simulink model "Perfect_Lineaer"  (R2017a)
settings: Solver=VariableStepAuto  StartTime=0.0  StopTime=17  FixedStep=0.01  RelTol=1e-3
values from neighbouring files (symbols this model uses):
  A = [-4.65E-06	0.0001701	-0.0002836	0	0	0	-2.56E-06	-7.97E-06	3.61E-06 ... (first row only)    [surfaces_setup_test.m]
  A0 = [-4.65E-06	0.0001701	-0.0002836	0	0	0	0	-1.43	0 ... (first row only)    [surfaces_setup_test.m]
  a0_s2345 = [0;0;0.05;0.05]    [HW5_4_surfaces.m]    (also in TEST_aerosetup.m; surfaces_setup_test.m)
  A_2345 = c_2345.*b_2345    [HW5_4_surfaces.m]    (also in TEST_aerosetup.m; surfaces_setup_test.m)
  Aileron_left = 0    [HW5_4_surfaces.m]    (also in TEST_aerosetup.m; surfaces_setup_test.m)
  Aileron_right = 0    [HW5_4_surfaces.m]    (also in TEST_aerosetup.m; surfaces_setup_test.m)
  B = [-7.98E-09	7.83E-09	1.68E-09	2.75E-10 ... (first row only)    [surfaces_setup_test.m]
  B0 = [-6.2	6.2	0	0.45 ... (first row only)    [surfaces_setup_test.m]
  c_2345 = [0.075;0.08;0.1;0.1]    [HW5_4_surfaces.m]    (also in TEST_aerosetup.m; surfaces_setup_test.m)
  CD0_s2345 = [0.01;0.01;0.01;0.01]    [HW5_4_surfaces.m]    (also in TEST_aerosetup.m; surfaces_setup_test.m)
  CDa_s2345 = [1;1;1;1]    [HW5_4_surfaces.m]    (also in TEST_aerosetup.m; surfaces_setup_test.m)
  CL0_2345 = [0;0; 0.05; 0.05]    [HW5_4_surfaces.m]    (also in TEST_aerosetup.m; surfaces_setup_test.m)
  CLa = 2*pi*(r./(2+r))    [HW5_4_surfaces.m]    (also in TEST_aerosetup.m; surfaces_setup_test.m)
  CM0_s2345 = [0;0;-0.05;-0.05]    [HW5_4_surfaces.m]    (also in TEST_aerosetup.m; surfaces_setup_test.m)
  CMa_s2345 = [0; 0; 0; 0]    [HW5_4_surfaces.m]    (also in TEST_aerosetup.m; surfaces_setup_test.m)
  e_s2345 = [0.8;0.8;0.9;0.9]    [HW5_4_surfaces.m]    (also in TEST_aerosetup.m; surfaces_setup_test.m)
  elevator = 0    [HW5_4_surfaces.m]    (also in TEST_aerosetup.m; surfaces_setup_test.m)
  Fext_N = -g_EN * m    [HW5_4_surfaces.m]    (also in TEST_aerosetup.m = [10 10 10]; surfaces_setup_test.m)
  g_EN = [0; 0; 9.81]    [HW5_4_surfaces.m]    (also in TEST_aerosetup.m = [0; 0; 9.8]; surfaces_setup_test.m)
  i_s2345 = [0; 0; 0.05; 0.05;]    [HW5_4_surfaces.m]    (also in TEST_aerosetup.m; surfaces_setup_test.m)
  J_cgp = ones(3)    [surfaces_setup_test.m]
  M_total = sum(MnG(:,1))/1000    [HW5_4_surfaces.m]    (also in TEST_aerosetup.m; surfaces_setup_test.m = sum(MnG1(:,1))/1000)
  Mext_B = [0; 0; 0]    [HW5_4_surfaces.m]    (also in TEST_aerosetup.m = [1; 1; 1]; surfaces_setup_test.m)
  p_E_BE_ini = p_E_BE_ini_deg .* [deg2rad; deg2rad; 1]    [HW5_4_surfaces.m]    (also in TEST_aerosetup.m; surfaces_setup_test.m)
  r = b_2345./c_2345    [HW5_4_surfaces.m]    (also in TEST_aerosetup.m; surfaces_setup_test.m)
  Rearth = 6371000    [HW5_4_surfaces.m]    (also in TEST_aerosetup.m; surfaces_setup_test.m)
  rudder = 0    [HW5_4_surfaces.m]    (also in TEST_aerosetup.m; surfaces_setup_test.m)
  Theta_ini = Theta_ini_deg * deg2rad    [HW5_4_surfaces.m]    (also in TEST_aerosetup.m; surfaces_setup_test.m)
  U0 = [Aileron_right;Aileron_left;elevator;rudder]    [surfaces_setup_test.m]
  v_N_AE = [0;0;0]    [HW5_4_surfaces.m]    (also in TEST_aerosetup.m; surfaces_setup_test.m)
  Vbbe_int = [10; 0; 0]    [HW5_4_surfaces.m]    (also in TEST_aerosetup.m; surfaces_setup_test.m = [5; 0; 0])
  w_B_BE_ini = [1e0; 1e-2; 1e-2]    [HW5_4_surfaces.m]    (also in TEST_aerosetup.m; surfaces_setup_test.m)
  X0 = [w_B_BE_ini;Theta_ini;Vbbe_int]    [surfaces_setup_test.m]
  xyz_s = [[-0.76 0 0.16];[-0.76 0 -0.09];[-0.23 0.44 0];[-0.23 -0.44 0];]    [HW5_4_surfaces.m]    (also in TEST_aerosetup.m; surfaces_setup_test.m)
undefined symbols (not defined in the file or in its folder): Discrete, Earth, K, Time, WGS84
libraries: simulink x83, aerolibfltsims x5, dspsrcs4 x4, simulink_extras x4, dspinverses x3, vrlib x2, sharedtransform x1, aerolibtransform2 x1, aerolibutil x1, sharedutil x1, ctrlSharedLib x1
(part 3 of 8)

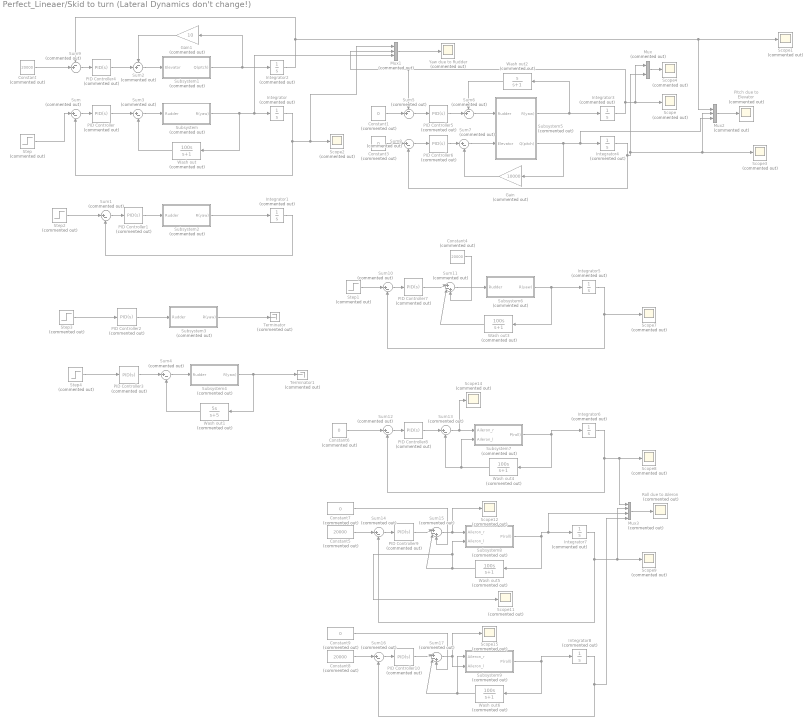
== system Perfect_Lineaer/Skid to turn (Lateral Dynamics don't change!) ==
  Constant{,4..5,8} (4 alike) : Constant  Commented=on  Value=20000
  Constant{1,3,6..7,9} (5 alike) : Constant  Commented=on  Value=0
  Gain : Gain  Commented=on  Gain=10000
  Gain1 : Gain  Commented=on  Gain=10
  Integrator{,1..8} (9 alike) : Integrator  Commented=on
  Mux : Mux  Commented=on  Inputs=2
  Mux1 : Mux  Commented=on  Inputs=3
  Mux2 : Mux  Commented=on  Inputs=3
  Mux3 : Mux  Commented=on
  PID Controller : simulink/Continuous/PID Controller  Commented=on  Controller=PID  TimeDomain=Continuous-time  SampleTime=-1  IntegratorMethod=Forward Euler  FilterMethod=Forward Euler  Form=Parallel  UseFilter=on  ControllerParametersSource=internal  P=1000  I=0  D=1  N=100  InitialConditionSource=internal  InitialConditionForIntegrator=0  InitialConditionForFilter=0  ExternalReset=none  LimitOutput=off  UpperSaturationLimit=inf  LowerSaturationLimit=-inf  LinearizeAsGain=on  AntiWindupMode=none  Kb=1  TrackingMode=off  Kt=1  PParamMin=[]  PParamMax=[]  IParamMin=[]  IParamMax=[]  DParamMin=[]  DParamMax=[]  NParamMin=[]  NParamMax=[]  KbParamMin=[]  KbParamMax=[]  KtParamMin=[]  KtParamMax=[]  POutMin=[]  POutMax=[]  IOutMin=[]  IOutMax=[]  DOutMin=[]  DOutMax=[]  NOutMin=[]  NOutMax=[]  KbOutMin=[]  KbOutMax=[]  KtOutMin=[]  KtOutMax=[]  IntegratorOutMin=[]  IntegratorOutMax=[]  FilterOutMin=[]  FilterOutMax=[]  SumOutMin=[]  SumOutMax=[]  SumI1OutMin=[]  SumI1OutMax=[]  SumI2OutMin=[]  SumI2OutMax=[]  SumI3OutMin=[]  SumI3OutMax=[]  SumDOutMin=[]  SumDOutMax=[]  SaturationOutMin=[]  SaturationOutMax=[]  IntegratorContinuousStateAttributes=''  IntegratorStateMustResolveToSignalObject=off  IntegratorRTWStateStorageClass=Auto  FilterContinuousStateAttributes=''  FilterStateMustResolveToSignalObject=off  FilterRTWStateStorageClass=Auto  DifferentiatorICPrevScaledInput=0  DifferentiatorOutMin=[]  DifferentiatorOutMax=[]  InitialConditionSetting=State (most efficient)
  PID Controller1 : simulink/Continuous/PID Controller  Commented=on  Controller=PID  TimeDomain=Continuous-time  SampleTime=-1  IntegratorMethod=Forward Euler  FilterMethod=Forward Euler  Form=Parallel  UseFilter=on  ControllerParametersSource=internal  P=1  I=0  D=0  N=100  InitialConditionSource=internal  InitialConditionForIntegrator=0  InitialConditionForFilter=0  ExternalReset=none  LimitOutput=off  UpperSaturationLimit=inf  LowerSaturationLimit=-inf  LinearizeAsGain=on  AntiWindupMode=none  Kb=1  TrackingMode=off  Kt=1  PParamMin=[]  PParamMax=[]  IParamMin=[]  IParamMax=[]  DParamMin=[]  DParamMax=[]  NParamMin=[]  NParamMax=[]  KbParamMin=[]  KbParamMax=[]  KtParamMin=[]  KtParamMax=[]  POutMin=[]  POutMax=[]  IOutMin=[]  IOutMax=[]  DOutMin=[]  DOutMax=[]  NOutMin=[]  NOutMax=[]  KbOutMin=[]  KbOutMax=[]  KtOutMin=[]  KtOutMax=[]  IntegratorOutMin=[]  IntegratorOutMax=[]  FilterOutMin=[]  FilterOutMax=[]  SumOutMin=[]  SumOutMax=[]  SumI1OutMin=[]  SumI1OutMax=[]  SumI2OutMin=[]  SumI2OutMax=[]  SumI3OutMin=[]  SumI3OutMax=[]  SumDOutMin=[]  SumDOutMax=[]  SaturationOutMin=[]  SaturationOutMax=[]  IntegratorContinuousStateAttributes=''  IntegratorStateMustResolveToSignalObject=off  IntegratorRTWStateStorageClass=Auto  FilterContinuousStateAttributes=''  FilterStateMustResolveToSignalObject=off  FilterRTWStateStorageClass=Auto  DifferentiatorICPrevScaledInput=0  DifferentiatorOutMin=[]  DifferentiatorOutMax=[]  InitialConditionSetting=State (most efficient)
  PID Controller10 : simulink/Continuous/PID Controller  Commented=on  Controller=PID  TimeDomain=Continuous-time  SampleTime=-1  IntegratorMethod=Forward Euler  FilterMethod=Forward Euler  Form=Parallel  UseFilter=on  ControllerParametersSource=internal  P=1000  I=0  D=0  N=100  InitialConditionSource=internal  InitialConditionForIntegrator=0  InitialConditionForFilter=0  ExternalReset=none  LimitOutput=off  UpperSaturationLimit=inf  LowerSaturationLimit=-inf  LinearizeAsGain=on  AntiWindupMode=none  Kb=1  TrackingMode=off  Kt=1  PParamMin=[]  PParamMax=[]  IParamMin=[]  IParamMax=[]  DParamMin=[]  DParamMax=[]  NParamMin=[]  NParamMax=[]  KbParamMin=[]  KbParamMax=[]  KtParamMin=[]  KtParamMax=[]  POutMin=[]  POutMax=[]  IOutMin=[]  IOutMax=[]  DOutMin=[]  DOutMax=[]  NOutMin=[]  NOutMax=[]  KbOutMin=[]  KbOutMax=[]  KtOutMin=[]  KtOutMax=[]  IntegratorOutMin=[]  IntegratorOutMax=[]  FilterOutMin=[]  FilterOutMax=[]  SumOutMin=[]  SumOutMax=[]  SumI1OutMin=[]  SumI1OutMax=[]  SumI2OutMin=[]  SumI2OutMax=[]  SumI3OutMin=[]  SumI3OutMax=[]  SumDOutMin=[]  SumDOutMax=[]  SaturationOutMin=[]  SaturationOutMax=[]  IntegratorContinuousStateAttributes=''  IntegratorStateMustResolveToSignalObject=off  IntegratorRTWStateStorageClass=Auto  FilterContinuousStateAttributes=''  FilterStateMustResolveToSignalObject=off  FilterRTWStateStorageClass=Auto  DifferentiatorICPrevScaledInput=0  DifferentiatorOutMin=[]  DifferentiatorOutMax=[]  InitialConditionSetting=State (most efficient)
  PID Controller2 : simulink/Continuous/PID Controller  Commented=on  Controller=PID  TimeDomain=Continuous-time  SampleTime=-1  IntegratorMethod=Forward Euler  FilterMethod=Forward Euler  Form=Parallel  UseFilter=on  ControllerParametersSource=internal  P=1  I=0  D=0  N=100  InitialConditionSource=internal  InitialConditionForIntegrator=0  InitialConditionForFilter=0  ExternalReset=none  LimitOutput=off  UpperSaturationLimit=inf  LowerSaturationLimit=-inf  LinearizeAsGain=on  AntiWindupMode=none  Kb=1  TrackingMode=off  Kt=1  PParamMin=[]  PParamMax=[]  IParamMin=[]  IParamMax=[]  DParamMin=[]  DParamMax=[]  NParamMin=[]  NParamMax=[]  KbParamMin=[]  KbParamMax=[]  KtParamMin=[]  KtParamMax=[]  POutMin=[]  POutMax=[]  IOutMin=[]  IOutMax=[]  DOutMin=[]  DOutMax=[]  NOutMin=[]  NOutMax=[]  KbOutMin=[]  KbOutMax=[]  KtOutMin=[]  KtOutMax=[]  IntegratorOutMin=[]  IntegratorOutMax=[]  FilterOutMin=[]  FilterOutMax=[]  SumOutMin=[]  SumOutMax=[]  SumI1OutMin=[]  SumI1OutMax=[]  SumI2OutMin=[]  SumI2OutMax=[]  SumI3OutMin=[]  SumI3OutMax=[]  SumDOutMin=[]  SumDOutMax=[]  SaturationOutMin=[]  SaturationOutMax=[]  IntegratorContinuousStateAttributes=''  IntegratorStateMustResolveToSignalObject=off  IntegratorRTWStateStorageClass=Auto  FilterContinuousStateAttributes=''  FilterStateMustResolveToSignalObject=off  FilterRTWStateStorageClass=Auto  DifferentiatorICPrevScaledInput=0  DifferentiatorOutMin=[]  DifferentiatorOutMax=[]  InitialConditionSetting=State (most efficient)
  PID Controller3 : simulink/Continuous/PID Controller  Commented=on  Controller=PID  TimeDomain=Continuous-time  SampleTime=-1  IntegratorMethod=Forward Euler  FilterMethod=Forward Euler  Form=Parallel  UseFilter=on  ControllerParametersSource=internal  P=1  I=0  D=0  N=100  InitialConditionSource=internal  InitialConditionForIntegrator=0  InitialConditionForFilter=0  ExternalReset=none  LimitOutput=off  UpperSaturationLimit=inf  LowerSaturationLimit=-inf  LinearizeAsGain=on  AntiWindupMode=none  Kb=1  TrackingMode=off  Kt=1  PParamMin=[]  PParamMax=[]  IParamMin=[]  IParamMax=[]  DParamMin=[]  DParamMax=[]  NParamMin=[]  NParamMax=[]  KbParamMin=[]  KbParamMax=[]  KtParamMin=[]  KtParamMax=[]  POutMin=[]  POutMax=[]  IOutMin=[]  IOutMax=[]  DOutMin=[]  DOutMax=[]  NOutMin=[]  NOutMax=[]  KbOutMin=[]  KbOutMax=[]  KtOutMin=[]  KtOutMax=[]  IntegratorOutMin=[]  IntegratorOutMax=[]  FilterOutMin=[]  FilterOutMax=[]  SumOutMin=[]  SumOutMax=[]  SumI1OutMin=[]  SumI1OutMax=[]  SumI2OutMin=[]  SumI2OutMax=[]  SumI3OutMin=[]  SumI3OutMax=[]  SumDOutMin=[]  SumDOutMax=[]  SaturationOutMin=[]  SaturationOutMax=[]  IntegratorContinuousStateAttributes=''  IntegratorStateMustResolveToSignalObject=off  IntegratorRTWStateStorageClass=Auto  FilterContinuousStateAttributes=''  FilterStateMustResolveToSignalObject=off  FilterRTWStateStorageClass=Auto  DifferentiatorICPrevScaledInput=0  DifferentiatorOutMin=[]  DifferentiatorOutMax=[]  InitialConditionSetting=State (most efficient)
  PID Controller4 : simulink/Continuous/PID Controller  Commented=on  Controller=PID  TimeDomain=Continuous-time  SampleTime=-1  IntegratorMethod=Forward Euler  FilterMethod=Forward Euler  Form=Parallel  UseFilter=on  ControllerParametersSource=internal  P=1000  I=0  D=0  N=100  InitialConditionSource=internal  InitialConditionForIntegrator=0  InitialConditionForFilter=0  ExternalReset=none  LimitOutput=off  UpperSaturationLimit=inf  LowerSaturationLimit=-inf  LinearizeAsGain=on  AntiWindupMode=none  Kb=1  TrackingMode=off  Kt=1  PParamMin=[]  PParamMax=[]  IParamMin=[]  IParamMax=[]  DParamMin=[]  DParamMax=[]  NParamMin=[]  NParamMax=[]  KbParamMin=[]  KbParamMax=[]  KtParamMin=[]  KtParamMax=[]  POutMin=[]  POutMax=[]  IOutMin=[]  IOutMax=[]  DOutMin=[]  DOutMax=[]  NOutMin=[]  NOutMax=[]  KbOutMin=[]  KbOutMax=[]  KtOutMin=[]  KtOutMax=[]  IntegratorOutMin=[]  IntegratorOutMax=[]  FilterOutMin=[]  FilterOutMax=[]  SumOutMin=[]  SumOutMax=[]  SumI1OutMin=[]  SumI1OutMax=[]  SumI2OutMin=[]  SumI2OutMax=[]  SumI3OutMin=[]  SumI3OutMax=[]  SumDOutMin=[]  SumDOutMax=[]  SaturationOutMin=[]  SaturationOutMax=[]  IntegratorContinuousStateAttributes=''  IntegratorStateMustResolveToSignalObject=off  IntegratorRTWStateStorageClass=Auto  FilterContinuousStateAttributes=''  FilterStateMustResolveToSignalObject=off  FilterRTWStateStorageClass=Auto  DifferentiatorICPrevScaledInput=0  DifferentiatorOutMin=[]  DifferentiatorOutMax=[]  InitialConditionSetting=State (most efficient)
  PID Controller5 : simulink/Continuous/PID Controller  Commented=on  Controller=PID  TimeDomain=Continuous-time  SampleTime=-1  IntegratorMethod=Forward Euler  FilterMethod=Forward Euler  Form=Parallel  UseFilter=on  ControllerParametersSource=internal  P=1000  I=0  D=1  N=100  InitialConditionSource=internal  InitialConditionForIntegrator=0  InitialConditionForFilter=0  ExternalReset=none  LimitOutput=off  UpperSaturationLimit=inf  LowerSaturationLimit=-inf  LinearizeAsGain=on  AntiWindupMode=none  Kb=1  TrackingMode=off  Kt=1  PParamMin=[]  PParamMax=[]  IParamMin=[]  IParamMax=[]  DParamMin=[]  DParamMax=[]  NParamMin=[]  NParamMax=[]  KbParamMin=[]  KbParamMax=[]  KtParamMin=[]  KtParamMax=[]  POutMin=[]  POutMax=[]  IOutMin=[]  IOutMax=[]  DOutMin=[]  DOutMax=[]  NOutMin=[]  NOutMax=[]  KbOutMin=[]  KbOutMax=[]  KtOutMin=[]  KtOutMax=[]  IntegratorOutMin=[]  IntegratorOutMax=[]  FilterOutMin=[]  FilterOutMax=[]  SumOutMin=[]  SumOutMax=[]  SumI1OutMin=[]  SumI1OutMax=[]  SumI2OutMin=[]  SumI2OutMax=[]  SumI3OutMin=[]  SumI3OutMax=[]  SumDOutMin=[]  SumDOutMax=[]  SaturationOutMin=[]  SaturationOutMax=[]  IntegratorContinuousStateAttributes=''  IntegratorStateMustResolveToSignalObject=off  IntegratorRTWStateStorageClass=Auto  FilterContinuousStateAttributes=''  FilterStateMustResolveToSignalObject=off  FilterRTWStateStorageClass=Auto  DifferentiatorICPrevScaledInput=0  DifferentiatorOutMin=[]  DifferentiatorOutMax=[]  InitialConditionSetting=State (most efficient)
  PID Controller6 : simulink/Continuous/PID Controller  Commented=on  Controller=PID  TimeDomain=Continuous-time  SampleTime=-1  IntegratorMethod=Forward Euler  FilterMethod=Forward Euler  Form=Parallel  UseFilter=on  ControllerParametersSource=internal  P=1000  I=0  D=0  N=100  InitialConditionSource=internal  InitialConditionForIntegrator=0  InitialConditionForFilter=0  ExternalReset=none  LimitOutput=off  UpperSaturationLimit=inf  LowerSaturationLimit=-inf  LinearizeAsGain=on  AntiWindupMode=none  Kb=1  TrackingMode=off  Kt=1  PParamMin=[]  PParamMax=[]  IParamMin=[]  IParamMax=[]  DParamMin=[]  DParamMax=[]  NParamMin=[]  NParamMax=[]  KbParamMin=[]  KbParamMax=[]  KtParamMin=[]  KtParamMax=[]  POutMin=[]  POutMax=[]  IOutMin=[]  IOutMax=[]  DOutMin=[]  DOutMax=[]  NOutMin=[]  NOutMax=[]  KbOutMin=[]  KbOutMax=[]  KtOutMin=[]  KtOutMax=[]  IntegratorOutMin=[]  IntegratorOutMax=[]  FilterOutMin=[]  FilterOutMax=[]  SumOutMin=[]  SumOutMax=[]  SumI1OutMin=[]  SumI1OutMax=[]  SumI2OutMin=[]  SumI2OutMax=[]  SumI3OutMin=[]  SumI3OutMax=[]  SumDOutMin=[]  SumDOutMax=[]  SaturationOutMin=[]  SaturationOutMax=[]  IntegratorContinuousStateAttributes=''  IntegratorStateMustResolveToSignalObject=off  IntegratorRTWStateStorageClass=Auto  FilterContinuousStateAttributes=''  FilterStateMustResolveToSignalObject=off  FilterRTWStateStorageClass=Auto  DifferentiatorICPrevScaledInput=0  DifferentiatorOutMin=[]  DifferentiatorOutMax=[]  InitialConditionSetting=State (most efficient)
  PID Controller7 : simulink/Continuous/PID Controller  Commented=on  Controller=PID  TimeDomain=Continuous-time  SampleTime=-1  IntegratorMethod=Forward Euler  FilterMethod=Forward Euler  Form=Parallel  UseFilter=on  ControllerParametersSource=internal  P=1  I=0  D=1  N=100  InitialConditionSource=internal  InitialConditionForIntegrator=0  InitialConditionForFilter=0  ExternalReset=none  LimitOutput=off  UpperSaturationLimit=inf  LowerSaturationLimit=-inf  LinearizeAsGain=on  AntiWindupMode=none  Kb=1  TrackingMode=off  Kt=1  PParamMin=[]  PParamMax=[]  IParamMin=[]  IParamMax=[]  DParamMin=[]  DParamMax=[]  NParamMin=[]  NParamMax=[]  KbParamMin=[]  KbParamMax=[]  KtParamMin=[]  KtParamMax=[]  POutMin=[]  POutMax=[]  IOutMin=[]  IOutMax=[]  DOutMin=[]  DOutMax=[]  NOutMin=[]  NOutMax=[]  KbOutMin=[]  KbOutMax=[]  KtOutMin=[]  KtOutMax=[]  IntegratorOutMin=[]  IntegratorOutMax=[]  FilterOutMin=[]  FilterOutMax=[]  SumOutMin=[]  SumOutMax=[]  SumI1OutMin=[]  SumI1OutMax=[]  SumI2OutMin=[]  SumI2OutMax=[]  SumI3OutMin=[]  SumI3OutMax=[]  SumDOutMin=[]  SumDOutMax=[]  SaturationOutMin=[]  SaturationOutMax=[]  IntegratorContinuousStateAttributes=''  IntegratorStateMustResolveToSignalObject=off  IntegratorRTWStateStorageClass=Auto  FilterContinuousStateAttributes=''  FilterStateMustResolveToSignalObject=off  FilterRTWStateStorageClass=Auto  DifferentiatorICPrevScaledInput=0  DifferentiatorOutMin=[]  DifferentiatorOutMax=[]  InitialConditionSetting=State (most efficient)
  PID Controller8 : simulink/Continuous/PID Controller  Commented=on  Controller=PID  TimeDomain=Continuous-time  SampleTime=-1  IntegratorMethod=Forward Euler  FilterMethod=Forward Euler  Form=Parallel  UseFilter=on  ControllerParametersSource=internal  P=10000  I=0  D=0  N=100  InitialConditionSource=internal  InitialConditionForIntegrator=0  InitialConditionForFilter=0  ExternalReset=none  LimitOutput=off  UpperSaturationLimit=inf  LowerSaturationLimit=-inf  LinearizeAsGain=on  AntiWindupMode=none  Kb=1  TrackingMode=off  Kt=1  PParamMin=[]  PParamMax=[]  IParamMin=[]  IParamMax=[]  DParamMin=[]  DParamMax=[]  NParamMin=[]  NParamMax=[]  KbParamMin=[]  KbParamMax=[]  KtParamMin=[]  KtParamMax=[]  POutMin=[]  POutMax=[]  IOutMin=[]  IOutMax=[]  DOutMin=[]  DOutMax=[]  NOutMin=[]  NOutMax=[]  KbOutMin=[]  KbOutMax=[]  KtOutMin=[]  KtOutMax=[]  IntegratorOutMin=[]  IntegratorOutMax=[]  FilterOutMin=[]  FilterOutMax=[]  SumOutMin=[]  SumOutMax=[]  SumI1OutMin=[]  SumI1OutMax=[]  SumI2OutMin=[]  SumI2OutMax=[]  SumI3OutMin=[]  SumI3OutMax=[]  SumDOutMin=[]  SumDOutMax=[]  SaturationOutMin=[]  SaturationOutMax=[]  IntegratorContinuousStateAttributes=''  IntegratorStateMustResolveToSignalObject=off  IntegratorRTWStateStorageClass=Auto  FilterContinuousStateAttributes=''  FilterStateMustResolveToSignalObject=off  FilterRTWStateStorageClass=Auto  DifferentiatorICPrevScaledInput=0  DifferentiatorOutMin=[]  DifferentiatorOutMax=[]  InitialConditionSetting=State (most efficient)
  PID Controller9 : simulink/Continuous/PID Controller  Commented=on  Controller=PID  TimeDomain=Continuous-time  SampleTime=-1  IntegratorMethod=Forward Euler  FilterMethod=Forward Euler  Form=Parallel  UseFilter=on  ControllerParametersSource=internal  P=100  I=0  D=0  N=100  InitialConditionSource=internal  InitialConditionForIntegrator=0  InitialConditionForFilter=0  ExternalReset=none  LimitOutput=off  UpperSaturationLimit=inf  LowerSaturationLimit=-inf  LinearizeAsGain=on  AntiWindupMode=none  Kb=1  TrackingMode=off  Kt=1  PParamMin=[]  PParamMax=[]  IParamMin=[]  IParamMax=[]  DParamMin=[]  DParamMax=[]  NParamMin=[]  NParamMax=[]  KbParamMin=[]  KbParamMax=[]  KtParamMin=[]  KtParamMax=[]  POutMin=[]  POutMax=[]  IOutMin=[]  IOutMax=[]  DOutMin=[]  DOutMax=[]  NOutMin=[]  NOutMax=[]  KbOutMin=[]  KbOutMax=[]  KtOutMin=[]  KtOutMax=[]  IntegratorOutMin=[]  IntegratorOutMax=[]  FilterOutMin=[]  FilterOutMax=[]  SumOutMin=[]  SumOutMax=[]  SumI1OutMin=[]  SumI1OutMax=[]  SumI2OutMin=[]  SumI2OutMax=[]  SumI3OutMin=[]  SumI3OutMax=[]  SumDOutMin=[]  SumDOutMax=[]  SaturationOutMin=[]  SaturationOutMax=[]  IntegratorContinuousStateAttributes=''  IntegratorStateMustResolveToSignalObject=off  IntegratorRTWStateStorageClass=Auto  FilterContinuousStateAttributes=''  FilterStateMustResolveToSignalObject=off  FilterRTWStateStorageClass=Auto  DifferentiatorICPrevScaledInput=0  DifferentiatorOutMin=[]  DifferentiatorOutMax=[]  InitialConditionSetting=State (most efficient)
  Pitch due to Elevator : Scope  Commented=on
  Roll due to Aileron : Scope  Commented=on
  Scope{,1..4,7..9,11..12,14..15} (12 alike) : Scope  Commented=on
  Step : Step  Commented=on  After=-20000  SampleTime=0
  Step1 : Step  Commented=on  After=-20000  SampleTime=0
  Step2 : Step  Commented=on  Time=0  After=0.000001  SampleTime=0
  Step3 : Step  Commented=on  Time=5  After=10  SampleTime=0
  Step4 : Step  Commented=on  Time=5  After=10  SampleTime=0
  Subsystem : Subsystem  Commented=on
  Subsystem1 : Subsystem  Commented=on
  Subsystem2 : Subsystem  Commented=on
  Subsystem3 : Subsystem  Commented=on
  Subsystem4 : Subsystem  Commented=on
  Subsystem5 : Subsystem  Commented=on
  Subsystem6 : Subsystem  Commented=on
  Subsystem7 : Subsystem  Commented=on
  Subsystem8 : Subsystem  Commented=on
  Subsystem9 : Subsystem  Commented=on
  Sum{,1,3..4,7..8,10,12..14,16} (11 alike) : Sum  Commented=on  Inputs=|+-
  Sum11 : Sum  Commented=on  Inputs=|+-+
  Sum15 : Sum  Commented=on  Inputs=|+-+
  Sum17 : Sum  Commented=on  Inputs=|+-+
  Sum{2,5..6,9} (4 alike) : Sum  Commented=on  Inputs=-+|
  Terminator : Terminator  Commented=on
  Terminator1 : Terminator  Commented=on
  Wash out{,3..6} (5 alike) : TransferFcn  Commented=on  Numerator=[100 0]  Denominator=[1 1]
  Wash out1 : TransferFcn  Commented=on  Numerator=[5 0]  Denominator=[1 5]
  Wash out2 : TransferFcn  Commented=on  Numerator=[1 0]  Denominator=[1 1]
  Yaw due to Rudder : Scope  Commented=on
  wires:
  Sum/1 -> PID Controller/1
  Subsystem/1(R(yaw)) -> Wash out/1, Mux1/3, Integrator/1
  Integrator/1 -> Sum/2, Mux1/1, Scope2/1
  Subsystem2/1(R(yaw)) -> Integrator1/1
  Step2/1 -> Sum1/1
  Sum1/1 -> PID Controller1/1
  PID Controller1/1 -> Subsystem2/1(Rudder)
  Integrator1/1 -> Sum1/2
  Subsystem3/1(R(yaw)) -> Terminator/1
  Step3/1 -> PID Controller2/1
  PID Controller2/1 -> Subsystem3/1(Rudder)
  Wash out/1 -> Sum3/2
  PID Controller/1 -> Sum3/1
  Sum3/1 -> Subsystem/1(Rudder)
  Subsystem4/1(R(yaw)) -> Terminator1/1, Wash out1/1
  PID Controller3/1 -> Sum4/1
  Wash out1/1 -> Sum4/2
  Sum4/1 -> Subsystem4/1(Rudder)
  Step4/1 -> PID Controller3/1
  Sum6/1 -> Subsystem5/1(Rudder)
  Subsystem5/1(R(yaw)) -> Wash out2/1, Integrator3/1
  Constant1/1 -> Sum5/2
  PID Controller5/1 -> Sum6/2
  Wash out2/1 -> Sum6/1
  Subsystem5/2(Q(pitch)) -> Gain/1, Mux2/3, Integrator4/1
  Sum5/1 -> PID Controller5/1
  Integrator3/1 -> Mux/1, Scope/1, Mux1/2, Sum5/1
  PID Controller6/1 -> Sum7/1
  Sum7/1 -> Subsystem5/2(Elevator)
  Sum8/1 -> PID Controller6/1
  Gain/1 -> Sum7/2
  Subsystem1/1(Q(pitch)) -> Gain1/1, Integrator2/1
  PID Controller4/1 -> Sum2/2
  Sum2/1 -> Subsystem1/1(Elevator)
  Sum9/1 -> PID Controller4/1
  Constant/1 -> Sum9/2
  Integrator2/1 -> Sum9/1, Mux2/1, Scope1/1
  Gain1/1 -> Sum2/1
  Integrator4/1 -> Sum8/2, Mux2/2, Scope3/1, Mux/2
  Mux/1 -> Scope4/1
  Mux1/1 -> Yaw due to Rudder/1
  Mux2/1 -> Pitch due to Elevator/1
  Constant3/1 -> Sum8/1
  Step/1 -> Sum/1
  Step1/1 -> Sum10/1
  Sum11/1 -> Subsystem6/1(Rudder)
  PID Controller7/1 -> Sum11/1
  Wash out3/1 -> Sum11/2
  Subsystem6/1(R(yaw)) -> Wash out3/1, Integrator5/1
  Integrator5/1 -> Sum10/2, Scope7/1
  Sum10/1 -> PID Controller7/1
  Constant6/1 -> Sum12/1
  Sum13/1 -> Scope14/1, Subsystem7/1(Aileron_r)
  PID Controller8/1 -> Sum13/1
  Subsystem7/1(P(roll)) -> Wash out4/1, Integrator6/1
  Integrator6/1 -> Sum12/2, Mux3/1, Scope8/1
  Sum12/1 -> PID Controller8/1
  Integrator7/1 -> Sum14/2, Scope9/1, Mux3/2
  Subsystem8/1(P(roll)) -> Mux3/3, Integrator7/1, Wash out5/1
  Wash out5/1 -> Scope11/1, Subsystem8/2(Aileron_l), Sum15/2
  Sum15/1 -> Scope12/1, Subsystem8/1(Aileron_r)
  PID Controller9/1 -> Sum15/1
  Sum14/1 -> PID Controller9/1
  Constant5/1 -> Sum14/1
  Mux3/1 -> Roll due to Aileron/1
  Wash out4/1 -> Subsystem7/2(Aileron_l), Sum13/2
  Constant4/1 -> Sum11/3
  Constant7/1 -> Sum15/3
  Sum16/1 -> PID Controller10/1
  PID Controller10/1 -> Sum17/1
  Wash out6/1 -> Subsystem9/1(Aileron_r), Sum17/2
  Constant9/1 -> Sum17/3
  Integrator8/1 -> Mux3/4, Sum16/2
  Subsystem9/1(P(roll)) -> Integrator8/1, Wash out6/1
  Constant8/1 -> Sum16/1
  Sum17/1 -> Subsystem9/2(Aileron_l), Scope15/1

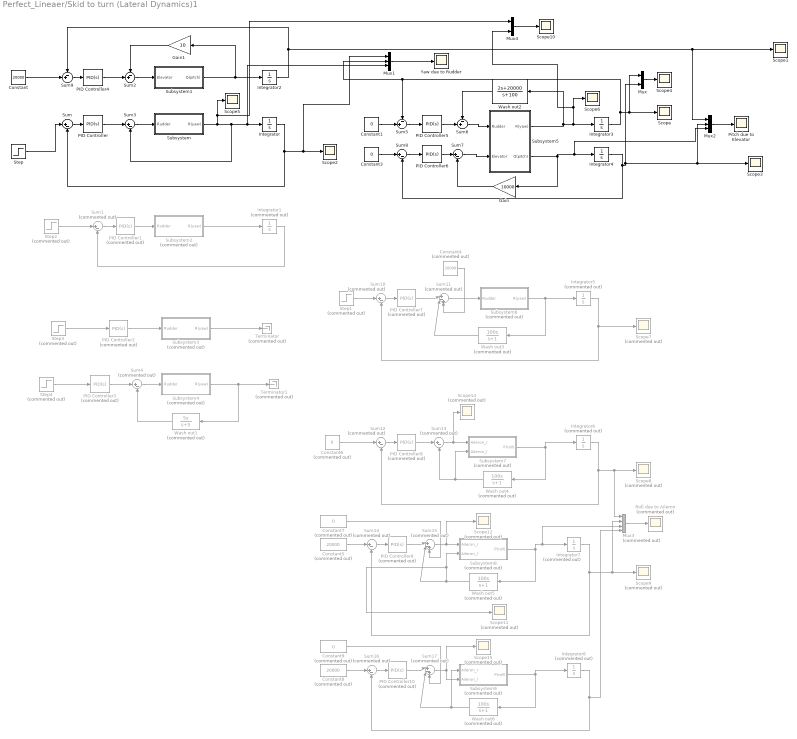
== system Perfect_Lineaer/Skid to turn (Lateral Dynamics)1 ==
  Constant : Constant  Value=20000
  Constant1 : Constant  Value=0
  Constant3 : Constant  Value=0
  Constant4 : Constant  Commented=on  Value=20000
  Constant5 : Constant  Commented=on  Value=20000
  Constant6 : Constant  Commented=on  Value=0
  Constant7 : Constant  Commented=on  Value=0
  Constant8 : Constant  Commented=on  Value=20000
  Constant9 : Constant  Commented=on  Value=0
  Gain : Gain  Gain=10000
  Gain1 : Gain  Gain=10
  Integrator{,2..4} (4 alike) : Integrator
  Integrator{1,5..8} (5 alike) : Integrator  Commented=on
  Mux : Mux  Inputs=2
  Mux1 : Mux  Inputs=3
  Mux2 : Mux  Inputs=3
  Mux3 : Mux  Commented=on
  Mux4 : Mux  Inputs=2
  PID Controller : simulink/Continuous/PID Controller  Controller=PID  TimeDomain=Continuous-time  SampleTime=-1  IntegratorMethod=Forward Euler  FilterMethod=Forward Euler  Form=Parallel  UseFilter=on  ControllerParametersSource=internal  P=1000000  I=0  D=1  N=100  InitialConditionSource=internal  InitialConditionForIntegrator=0  InitialConditionForFilter=0  ExternalReset=none  LimitOutput=off  UpperSaturationLimit=inf  LowerSaturationLimit=-inf  LinearizeAsGain=on  AntiWindupMode=none  Kb=1  TrackingMode=off  Kt=1  PParamMin=[]  PParamMax=[]  IParamMin=[]  IParamMax=[]  DParamMin=[]  DParamMax=[]  NParamMin=[]  NParamMax=[]  KbParamMin=[]  KbParamMax=[]  KtParamMin=[]  KtParamMax=[]  POutMin=[]  POutMax=[]  IOutMin=[]  IOutMax=[]  DOutMin=[]  DOutMax=[]  NOutMin=[]  NOutMax=[]  KbOutMin=[]  KbOutMax=[]  KtOutMin=[]  KtOutMax=[]  IntegratorOutMin=[]  IntegratorOutMax=[]  FilterOutMin=[]  FilterOutMax=[]  SumOutMin=[]  SumOutMax=[]  SumI1OutMin=[]  SumI1OutMax=[]  SumI2OutMin=[]  SumI2OutMax=[]  SumI3OutMin=[]  SumI3OutMax=[]  SumDOutMin=[]  SumDOutMax=[]  SaturationOutMin=[]  SaturationOutMax=[]  IntegratorContinuousStateAttributes=''  IntegratorStateMustResolveToSignalObject=off  IntegratorRTWStateStorageClass=Auto  FilterContinuousStateAttributes=''  FilterStateMustResolveToSignalObject=off  FilterRTWStateStorageClass=Auto  DifferentiatorICPrevScaledInput=0  DifferentiatorOutMin=[]  DifferentiatorOutMax=[]  InitialConditionSetting=State (most efficient)
  PID Controller1 : simulink/Continuous/PID Controller  Commented=on  Controller=PID  TimeDomain=Continuous-time  SampleTime=-1  IntegratorMethod=Forward Euler  FilterMethod=Forward Euler  Form=Parallel  UseFilter=on  ControllerParametersSource=internal  P=1  I=0  D=0  N=100  InitialConditionSource=internal  InitialConditionForIntegrator=0  InitialConditionForFilter=0  ExternalReset=none  LimitOutput=off  UpperSaturationLimit=inf  LowerSaturationLimit=-inf  LinearizeAsGain=on  AntiWindupMode=none  Kb=1  TrackingMode=off  Kt=1  PParamMin=[]  PParamMax=[]  IParamMin=[]  IParamMax=[]  DParamMin=[]  DParamMax=[]  NParamMin=[]  NParamMax=[]  KbParamMin=[]  KbParamMax=[]  KtParamMin=[]  KtParamMax=[]  POutMin=[]  POutMax=[]  IOutMin=[]  IOutMax=[]  DOutMin=[]  DOutMax=[]  NOutMin=[]  NOutMax=[]  KbOutMin=[]  KbOutMax=[]  KtOutMin=[]  KtOutMax=[]  IntegratorOutMin=[]  IntegratorOutMax=[]  FilterOutMin=[]  FilterOutMax=[]  SumOutMin=[]  SumOutMax=[]  SumI1OutMin=[]  SumI1OutMax=[]  SumI2OutMin=[]  SumI2OutMax=[]  SumI3OutMin=[]  SumI3OutMax=[]  SumDOutMin=[]  SumDOutMax=[]  SaturationOutMin=[]  SaturationOutMax=[]  IntegratorContinuousStateAttributes=''  IntegratorStateMustResolveToSignalObject=off  IntegratorRTWStateStorageClass=Auto  FilterContinuousStateAttributes=''  FilterStateMustResolveToSignalObject=off  FilterRTWStateStorageClass=Auto  DifferentiatorICPrevScaledInput=0  DifferentiatorOutMin=[]  DifferentiatorOutMax=[]  InitialConditionSetting=State (most efficient)
  PID Controller10 : simulink/Continuous/PID Controller  Commented=on  Controller=PID  TimeDomain=Continuous-time  SampleTime=-1  IntegratorMethod=Forward Euler  FilterMethod=Forward Euler  Form=Parallel  UseFilter=on  ControllerParametersSource=internal  P=1000  I=0  D=0  N=100  InitialConditionSource=internal  InitialConditionForIntegrator=0  InitialConditionForFilter=0  ExternalReset=none  LimitOutput=off  UpperSaturationLimit=inf  LowerSaturationLimit=-inf  LinearizeAsGain=on  AntiWindupMode=none  Kb=1  TrackingMode=off  Kt=1  PParamMin=[]  PParamMax=[]  IParamMin=[]  IParamMax=[]  DParamMin=[]  DParamMax=[]  NParamMin=[]  NParamMax=[]  KbParamMin=[]  KbParamMax=[]  KtParamMin=[]  KtParamMax=[]  POutMin=[]  POutMax=[]  IOutMin=[]  IOutMax=[]  DOutMin=[]  DOutMax=[]  NOutMin=[]  NOutMax=[]  KbOutMin=[]  KbOutMax=[]  KtOutMin=[]  KtOutMax=[]  IntegratorOutMin=[]  IntegratorOutMax=[]  FilterOutMin=[]  FilterOutMax=[]  SumOutMin=[]  SumOutMax=[]  SumI1OutMin=[]  SumI1OutMax=[]  SumI2OutMin=[]  SumI2OutMax=[]  SumI3OutMin=[]  SumI3OutMax=[]  SumDOutMin=[]  SumDOutMax=[]  SaturationOutMin=[]  SaturationOutMax=[]  IntegratorContinuousStateAttributes=''  IntegratorStateMustResolveToSignalObject=off  IntegratorRTWStateStorageClass=Auto  FilterContinuousStateAttributes=''  FilterStateMustResolveToSignalObject=off  FilterRTWStateStorageClass=Auto  DifferentiatorICPrevScaledInput=0  DifferentiatorOutMin=[]  DifferentiatorOutMax=[]  InitialConditionSetting=State (most efficient)
  PID Controller2 : simulink/Continuous/PID Controller  Commented=on  Controller=PID  TimeDomain=Continuous-time  SampleTime=-1  IntegratorMethod=Forward Euler  FilterMethod=Forward Euler  Form=Parallel  UseFilter=on  ControllerParametersSource=internal  P=1  I=0  D=0  N=100  InitialConditionSource=internal  InitialConditionForIntegrator=0  InitialConditionForFilter=0  ExternalReset=none  LimitOutput=off  UpperSaturationLimit=inf  LowerSaturationLimit=-inf  LinearizeAsGain=on  AntiWindupMode=none  Kb=1  TrackingMode=off  Kt=1  PParamMin=[]  PParamMax=[]  IParamMin=[]  IParamMax=[]  DParamMin=[]  DParamMax=[]  NParamMin=[]  NParamMax=[]  KbParamMin=[]  KbParamMax=[]  KtParamMin=[]  KtParamMax=[]  POutMin=[]  POutMax=[]  IOutMin=[]  IOutMax=[]  DOutMin=[]  DOutMax=[]  NOutMin=[]  NOutMax=[]  KbOutMin=[]  KbOutMax=[]  KtOutMin=[]  KtOutMax=[]  IntegratorOutMin=[]  IntegratorOutMax=[]  FilterOutMin=[]  FilterOutMax=[]  SumOutMin=[]  SumOutMax=[]  SumI1OutMin=[]  SumI1OutMax=[]  SumI2OutMin=[]  SumI2OutMax=[]  SumI3OutMin=[]  SumI3OutMax=[]  SumDOutMin=[]  SumDOutMax=[]  SaturationOutMin=[]  SaturationOutMax=[]  IntegratorContinuousStateAttributes=''  IntegratorStateMustResolveToSignalObject=off  IntegratorRTWStateStorageClass=Auto  FilterContinuousStateAttributes=''  FilterStateMustResolveToSignalObject=off  FilterRTWStateStorageClass=Auto  DifferentiatorICPrevScaledInput=0  DifferentiatorOutMin=[]  DifferentiatorOutMax=[]  InitialConditionSetting=State (most efficient)
  PID Controller3 : simulink/Continuous/PID Controller  Commented=on  Controller=PID  TimeDomain=Continuous-time  SampleTime=-1  IntegratorMethod=Forward Euler  FilterMethod=Forward Euler  Form=Parallel  UseFilter=on  ControllerParametersSource=internal  P=1  I=0  D=0  N=100  InitialConditionSource=internal  InitialConditionForIntegrator=0  InitialConditionForFilter=0  ExternalReset=none  LimitOutput=off  UpperSaturationLimit=inf  LowerSaturationLimit=-inf  LinearizeAsGain=on  AntiWindupMode=none  Kb=1  TrackingMode=off  Kt=1  PParamMin=[]  PParamMax=[]  IParamMin=[]  IParamMax=[]  DParamMin=[]  DParamMax=[]  NParamMin=[]  NParamMax=[]  KbParamMin=[]  KbParamMax=[]  KtParamMin=[]  KtParamMax=[]  POutMin=[]  POutMax=[]  IOutMin=[]  IOutMax=[]  DOutMin=[]  DOutMax=[]  NOutMin=[]  NOutMax=[]  KbOutMin=[]  KbOutMax=[]  KtOutMin=[]  KtOutMax=[]  IntegratorOutMin=[]  IntegratorOutMax=[]  FilterOutMin=[]  FilterOutMax=[]  SumOutMin=[]  SumOutMax=[]  SumI1OutMin=[]  SumI1OutMax=[]  SumI2OutMin=[]  SumI2OutMax=[]  SumI3OutMin=[]  SumI3OutMax=[]  SumDOutMin=[]  SumDOutMax=[]  SaturationOutMin=[]  SaturationOutMax=[]  IntegratorContinuousStateAttributes=''  IntegratorStateMustResolveToSignalObject=off  IntegratorRTWStateStorageClass=Auto  FilterContinuousStateAttributes=''  FilterStateMustResolveToSignalObject=off  FilterRTWStateStorageClass=Auto  DifferentiatorICPrevScaledInput=0  DifferentiatorOutMin=[]  DifferentiatorOutMax=[]  InitialConditionSetting=State (most efficient)
  PID Controller4 : simulink/Continuous/PID Controller  Controller=PID  TimeDomain=Continuous-time  SampleTime=-1  IntegratorMethod=Forward Euler  FilterMethod=Forward Euler  Form=Parallel  UseFilter=on  ControllerParametersSource=internal  P=1000  I=0  D=0  N=100  InitialConditionSource=internal  InitialConditionForIntegrator=0  InitialConditionForFilter=0  ExternalReset=none  LimitOutput=off  UpperSaturationLimit=inf  LowerSaturationLimit=-inf  LinearizeAsGain=on  AntiWindupMode=none  Kb=1  TrackingMode=off  Kt=1  PParamMin=[]  PParamMax=[]  IParamMin=[]  IParamMax=[]  DParamMin=[]  DParamMax=[]  NParamMin=[]  NParamMax=[]  KbParamMin=[]  KbParamMax=[]  KtParamMin=[]  KtParamMax=[]  POutMin=[]  POutMax=[]  IOutMin=[]  IOutMax=[]  DOutMin=[]  DOutMax=[]  NOutMin=[]  NOutMax=[]  KbOutMin=[]  KbOutMax=[]  KtOutMin=[]  KtOutMax=[]  IntegratorOutMin=[]  IntegratorOutMax=[]  FilterOutMin=[]  FilterOutMax=[]  SumOutMin=[]  SumOutMax=[]  SumI1OutMin=[]  SumI1OutMax=[]  SumI2OutMin=[]  SumI2OutMax=[]  SumI3OutMin=[]  SumI3OutMax=[]  SumDOutMin=[]  SumDOutMax=[]  SaturationOutMin=[]  SaturationOutMax=[]  IntegratorContinuousStateAttributes=''  IntegratorStateMustResolveToSignalObject=off  IntegratorRTWStateStorageClass=Auto  FilterContinuousStateAttributes=''  FilterStateMustResolveToSignalObject=off  FilterRTWStateStorageClass=Auto  DifferentiatorICPrevScaledInput=0  DifferentiatorOutMin=[]  DifferentiatorOutMax=[]  InitialConditionSetting=State (most efficient)
  PID Controller5 : simulink/Continuous/PID Controller  Controller=PID  TimeDomain=Continuous-time  SampleTime=-1  IntegratorMethod=Forward Euler  FilterMethod=Forward Euler  Form=Parallel  UseFilter=on  ControllerParametersSource=internal  P=1000  I=0  D=1  N=100  InitialConditionSource=internal  InitialConditionForIntegrator=0  InitialConditionForFilter=0  ExternalReset=none  LimitOutput=off  UpperSaturationLimit=inf  LowerSaturationLimit=-inf  LinearizeAsGain=on  AntiWindupMode=none  Kb=1  TrackingMode=off  Kt=1  PParamMin=[]  PParamMax=[]  IParamMin=[]  IParamMax=[]  DParamMin=[]  DParamMax=[]  NParamMin=[]  NParamMax=[]  KbParamMin=[]  KbParamMax=[]  KtParamMin=[]  KtParamMax=[]  POutMin=[]  POutMax=[]  IOutMin=[]  IOutMax=[]  DOutMin=[]  DOutMax=[]  NOutMin=[]  NOutMax=[]  KbOutMin=[]  KbOutMax=[]  KtOutMin=[]  KtOutMax=[]  IntegratorOutMin=[]  IntegratorOutMax=[]  FilterOutMin=[]  FilterOutMax=[]  SumOutMin=[]  SumOutMax=[]  SumI1OutMin=[]  SumI1OutMax=[]  SumI2OutMin=[]  SumI2OutMax=[]  SumI3OutMin=[]  SumI3OutMax=[]  SumDOutMin=[]  SumDOutMax=[]  SaturationOutMin=[]  SaturationOutMax=[]  IntegratorContinuousStateAttributes=''  IntegratorStateMustResolveToSignalObject=off  IntegratorRTWStateStorageClass=Auto  FilterContinuousStateAttributes=''  FilterStateMustResolveToSignalObject=off  FilterRTWStateStorageClass=Auto  DifferentiatorICPrevScaledInput=0  DifferentiatorOutMin=[]  DifferentiatorOutMax=[]  InitialConditionSetting=State (most efficient)
  PID Controller6 : simulink/Continuous/PID Controller  Controller=PID  TimeDomain=Continuous-time  SampleTime=-1  IntegratorMethod=Forward Euler  FilterMethod=Forward Euler  Form=Parallel  UseFilter=on  ControllerParametersSource=internal  P=1000  I=0  D=0  N=100  InitialConditionSource=internal  InitialConditionForIntegrator=0  InitialConditionForFilter=0  ExternalReset=none  LimitOutput=off  UpperSaturationLimit=inf  LowerSaturationLimit=-inf  LinearizeAsGain=on  AntiWindupMode=none  Kb=1  TrackingMode=off  Kt=1  PParamMin=[]  PParamMax=[]  IParamMin=[]  IParamMax=[]  DParamMin=[]  DParamMax=[]  NParamMin=[]  NParamMax=[]  KbParamMin=[]  KbParamMax=[]  KtParamMin=[]  KtParamMax=[]  POutMin=[]  POutMax=[]  IOutMin=[]  IOutMax=[]  DOutMin=[]  DOutMax=[]  NOutMin=[]  NOutMax=[]  KbOutMin=[]  KbOutMax=[]  KtOutMin=[]  KtOutMax=[]  IntegratorOutMin=[]  IntegratorOutMax=[]  FilterOutMin=[]  FilterOutMax=[]  SumOutMin=[]  SumOutMax=[]  SumI1OutMin=[]  SumI1OutMax=[]  SumI2OutMin=[]  SumI2OutMax=[]  SumI3OutMin=[]  SumI3OutMax=[]  SumDOutMin=[]  SumDOutMax=[]  SaturationOutMin=[]  SaturationOutMax=[]  IntegratorContinuousStateAttributes=''  IntegratorStateMustResolveToSignalObject=off  IntegratorRTWStateStorageClass=Auto  FilterContinuousStateAttributes=''  FilterStateMustResolveToSignalObject=off  FilterRTWStateStorageClass=Auto  DifferentiatorICPrevScaledInput=0  DifferentiatorOutMin=[]  DifferentiatorOutMax=[]  InitialConditionSetting=State (most efficient)
  PID Controller7 : simulink/Continuous/PID Controller  Commented=on  Controller=PID  TimeDomain=Continuous-time  SampleTime=-1  IntegratorMethod=Forward Euler  FilterMethod=Forward Euler  Form=Parallel  UseFilter=on  ControllerParametersSource=internal  P=1  I=0  D=1  N=100  InitialConditionSource=internal  InitialConditionForIntegrator=0  InitialConditionForFilter=0  ExternalReset=none  LimitOutput=off  UpperSaturationLimit=inf  LowerSaturationLimit=-inf  LinearizeAsGain=on  AntiWindupMode=none  Kb=1  TrackingMode=off  Kt=1  PParamMin=[]  PParamMax=[]  IParamMin=[]  IParamMax=[]  DParamMin=[]  DParamMax=[]  NParamMin=[]  NParamMax=[]  KbParamMin=[]  KbParamMax=[]  KtParamMin=[]  KtParamMax=[]  POutMin=[]  POutMax=[]  IOutMin=[]  IOutMax=[]  DOutMin=[]  DOutMax=[]  NOutMin=[]  NOutMax=[]  KbOutMin=[]  KbOutMax=[]  KtOutMin=[]  KtOutMax=[]  IntegratorOutMin=[]  IntegratorOutMax=[]  FilterOutMin=[]  FilterOutMax=[]  SumOutMin=[]  SumOutMax=[]  SumI1OutMin=[]  SumI1OutMax=[]  SumI2OutMin=[]  SumI2OutMax=[]  SumI3OutMin=[]  SumI3OutMax=[]  SumDOutMin=[]  SumDOutMax=[]  SaturationOutMin=[]  SaturationOutMax=[]  IntegratorContinuousStateAttributes=''  IntegratorStateMustResolveToSignalObject=off  IntegratorRTWStateStorageClass=Auto  FilterContinuousStateAttributes=''  FilterStateMustResolveToSignalObject=off  FilterRTWStateStorageClass=Auto  DifferentiatorICPrevScaledInput=0  DifferentiatorOutMin=[]  DifferentiatorOutMax=[]  InitialConditionSetting=State (most efficient)
  PID Controller8 : simulink/Continuous/PID Controller  Commented=on  Controller=PID  TimeDomain=Continuous-time  SampleTime=-1  IntegratorMethod=Forward Euler  FilterMethod=Forward Euler  Form=Parallel  UseFilter=on  ControllerParametersSource=internal  P=10000  I=0  D=0  N=100  InitialConditionSource=internal  InitialConditionForIntegrator=0  InitialConditionForFilter=0  ExternalReset=none  LimitOutput=off  UpperSaturationLimit=inf  LowerSaturationLimit=-inf  LinearizeAsGain=on  AntiWindupMode=none  Kb=1  TrackingMode=off  Kt=1  PParamMin=[]  PParamMax=[]  IParamMin=[]  IParamMax=[]  DParamMin=[]  DParamMax=[]  NParamMin=[]  NParamMax=[]  KbParamMin=[]  KbParamMax=[]  KtParamMin=[]  KtParamMax=[]  POutMin=[]  POutMax=[]  IOutMin=[]  IOutMax=[]  DOutMin=[]  DOutMax=[]  NOutMin=[]  NOutMax=[]  KbOutMin=[]  KbOutMax=[]  KtOutMin=[]  KtOutMax=[]  IntegratorOutMin=[]  IntegratorOutMax=[]  FilterOutMin=[]  FilterOutMax=[]  SumOutMin=[]  SumOutMax=[]  SumI1OutMin=[]  SumI1OutMax=[]  SumI2OutMin=[]  SumI2OutMax=[]  SumI3OutMin=[]  SumI3OutMax=[]  SumDOutMin=[]  SumDOutMax=[]  SaturationOutMin=[]  SaturationOutMax=[]  IntegratorContinuousStateAttributes=''  IntegratorStateMustResolveToSignalObject=off  IntegratorRTWStateStorageClass=Auto  FilterContinuousStateAttributes=''  FilterStateMustResolveToSignalObject=off  FilterRTWStateStorageClass=Auto  DifferentiatorICPrevScaledInput=0  DifferentiatorOutMin=[]  DifferentiatorOutMax=[]  InitialConditionSetting=State (most efficient)
  PID Controller9 : simulink/Continuous/PID Controller  Commented=on  Controller=PID  TimeDomain=Continuous-time  SampleTime=-1  IntegratorMethod=Forward Euler  FilterMethod=Forward Euler  Form=Parallel  UseFilter=on  ControllerParametersSource=internal  P=100  I=0  D=0  N=100  InitialConditionSource=internal  InitialConditionForIntegrator=0  InitialConditionForFilter=0  ExternalReset=none  LimitOutput=off  UpperSaturationLimit=inf  LowerSaturationLimit=-inf  LinearizeAsGain=on  AntiWindupMode=none  Kb=1  TrackingMode=off  Kt=1  PParamMin=[]  PParamMax=[]  IParamMin=[]  IParamMax=[]  DParamMin=[]  DParamMax=[]  NParamMin=[]  NParamMax=[]  KbParamMin=[]  KbParamMax=[]  KtParamMin=[]  KtParamMax=[]  POutMin=[]  POutMax=[]  IOutMin=[]  IOutMax=[]  DOutMin=[]  DOutMax=[]  NOutMin=[]  NOutMax=[]  KbOutMin=[]  KbOutMax=[]  KtOutMin=[]  KtOutMax=[]  IntegratorOutMin=[]  IntegratorOutMax=[]  FilterOutMin=[]  FilterOutMax=[]  SumOutMin=[]  SumOutMax=[]  SumI1OutMin=[]  SumI1OutMax=[]  SumI2OutMin=[]  SumI2OutMax=[]  SumI3OutMin=[]  SumI3OutMax=[]  SumDOutMin=[]  SumDOutMax=[]  SaturationOutMin=[]  SaturationOutMax=[]  IntegratorContinuousStateAttributes=''  IntegratorStateMustResolveToSignalObject=off  IntegratorRTWStateStorageClass=Auto  FilterContinuousStateAttributes=''  FilterStateMustResolveToSignalObject=off  FilterRTWStateStorageClass=Auto  DifferentiatorICPrevScaledInput=0  DifferentiatorOutMin=[]  DifferentiatorOutMax=[]  InitialConditionSetting=State (most efficient)
  Pitch due to Elevator : Scope
  Roll due to Aileron : Scope  Commented=on
  Scope{,1..6,10} (8 alike) : Scope
  Scope{7..9,11..12,14..15} (7 alike) : Scope  Commented=on
  Step : Step  After=0  SampleTime=0
  Step1 : Step  Commented=on  After=-20000  SampleTime=0
  Step2 : Step  Commented=on  Time=5  After=10  SampleTime=0
  Step3 : Step  Commented=on  Time=5  After=10  SampleTime=0
  Step4 : Step  Commented=on  Time=5  After=10  SampleTime=0
  Subsystem : Subsystem
  Subsystem1 : Subsystem
  Subsystem2 : Subsystem  Commented=on
  Subsystem3 : Subsystem  Commented=on
  Subsystem4 : Subsystem  Commented=on
  Subsystem5 : Subsystem
  Subsystem6 : Subsystem  Commented=on
  Subsystem7 : Subsystem  Commented=on
  Subsystem8 : Subsystem  Commented=on
  Subsystem9 : Subsystem  Commented=on
  Sum{,3,7..8} (4 alike) : Sum  Inputs=|+-
  Sum{1,4,10,12..14,16} (7 alike) : Sum  Commented=on  Inputs=|+-
  Sum11 : Sum  Commented=on  Inputs=|+-+
  Sum15 : Sum  Commented=on  Inputs=|+-+
  Sum17 : Sum  Commented=on  Inputs=|+-+
  Sum{2,5..6,9} (4 alike) : Sum  Inputs=-+|
  Terminator : Terminator  Commented=on
  Terminator1 : Terminator  Commented=on
  Wash out1 : TransferFcn  Commented=on  Numerator=[5 0]  Denominator=[1 5]
  Wash out2 : TransferFcn  Numerator=[2 20000]  Denominator=[1 100]
  Wash out{3..6} (4 alike) : TransferFcn  Commented=on  Numerator=[100 0]  Denominator=[1 1]
  Yaw due to Rudder : Scope
  wires:
  Sum/1 -> PID Controller/1
  Integrator/1 -> Sum/2, Mux1/1, Scope2/1
  Subsystem2/1(R(yaw)) -> Integrator1/1
  Step2/1 -> Sum1/1
  Sum1/1 -> PID Controller1/1
  PID Controller1/1 -> Subsystem2/1(Rudder)
  Integrator1/1 -> Sum1/2
  Subsystem3/1(R(yaw)) -> Terminator/1
  Step3/1 -> PID Controller2/1
  PID Controller2/1 -> Subsystem3/1(Rudder)
  Subsystem/1(R(yaw)) -> Mux4/1, Scope5/1, Sum3/2, Mux1/3, Integrator/1
  PID Controller/1 -> Sum3/1
  Sum3/1 -> Subsystem/1(Rudder)
  Subsystem4/1(R(yaw)) -> Terminator1/1, Wash out1/1
  PID Controller3/1 -> Sum4/1
  Wash out1/1 -> Sum4/2
  Sum4/1 -> Subsystem4/1(Rudder)
  Step4/1 -> PID Controller3/1
  Sum6/1 -> Subsystem5/1(Rudder)
  Subsystem5/1(R(yaw)) -> Wash out2/1, Mux4/2, Scope6/1, Integrator3/1
  Constant1/1 -> Sum5/2
  PID Controller5/1 -> Sum6/2
  Wash out2/1 -> Sum6/1
  Subsystem5/2(Q(pitch)) -> Mux2/3, Integrator4/1, Gain/1
  Sum5/1 -> PID Controller5/1
  Integrator3/1 -> Mux/1, Scope/1, Mux1/2, Sum5/1
  PID Controller6/1 -> Sum7/1
  Sum7/1 -> Subsystem5/2(Elevator)
  Sum8/1 -> PID Controller6/1
  Gain/1 -> Sum7/2
  Subsystem1/1(Q(pitch)) -> Gain1/1, Integrator2/1
  PID Controller4/1 -> Sum2/2
  Sum2/1 -> Subsystem1/1(Elevator)
  Sum9/1 -> PID Controller4/1
  Constant/1 -> Sum9/2
  Integrator2/1 -> Sum9/1, Mux2/1, Scope1/1
  Gain1/1 -> Sum2/1
  Integrator4/1 -> Sum8/2, Mux2/2, Scope3/1, Mux/2
  Mux/1 -> Scope4/1
  Mux1/1 -> Yaw due to Rudder/1
  Mux2/1 -> Pitch due to Elevator/1
  Constant3/1 -> Sum8/1
  Step/1 -> Sum/1
  Step1/1 -> Sum10/1
  Sum11/1 -> Subsystem6/1(Rudder)
  PID Controller7/1 -> Sum11/1
  Wash out3/1 -> Sum11/2
  Subsystem6/1(R(yaw)) -> Wash out3/1, Integrator5/1
  Integrator5/1 -> Sum10/2, Scope7/1
  Sum10/1 -> PID Controller7/1
  Constant6/1 -> Sum12/1
  Sum13/1 -> Scope14/1, Subsystem7/1(Aileron_r)
  PID Controller8/1 -> Sum13/1
  Subsystem7/1(P(roll)) -> Wash out4/1, Integrator6/1
  Integrator6/1 -> Sum12/2, Mux3/1, Scope8/1
  Sum12/1 -> PID Controller8/1
  Integrator7/1 -> Sum14/2, Scope9/1, Mux3/2
  Subsystem8/1(P(roll)) -> Mux3/3, Integrator7/1, Wash out5/1
  Wash out5/1 -> Scope11/1, Subsystem8/2(Aileron_l), Sum15/2
  Sum15/1 -> Scope12/1, Subsystem8/1(Aileron_r)
  PID Controller9/1 -> Sum15/1
  Sum14/1 -> PID Controller9/1
  Constant5/1 -> Sum14/1
  Mux3/1 -> Roll due to Aileron/1
  Wash out4/1 -> Subsystem7/2(Aileron_l), Sum13/2
  Constant4/1 -> Sum11/3
  Constant7/1 -> Sum15/3
  Sum16/1 -> PID Controller10/1
  PID Controller10/1 -> Sum17/1
  Wash out6/1 -> Subsystem9/1(Aileron_r), Sum17/2
  Constant9/1 -> Sum17/3
  Integrator8/1 -> Mux3/4, Sum16/2
  Subsystem9/1(P(roll)) -> Integrator8/1, Wash out6/1
  Constant8/1 -> Sum16/1
  Sum17/1 -> Subsystem9/2(Aileron_l), Scope15/1
  Mux4/1 -> Scope10/1
